simulink model "temp_regler"  (R2024a)
settings: Solver=VariableStepAuto  StartTime=0.0  StopTime=4200  RelTol=1e-3
values from neighbouring files (symbols this model uses):
  param_k1 = 10/400    (= 0.025)    [temp_regler.m]    (also in temp_regler_settings.m; temp_settings.m)
  param_k2 = 400/230    (= 1.73913043478)    [temp_regler.m]    (also in temp_regler_settings.m; temp_settings.m)
  param_switch_off = -0.2    [temp_regler.m]    (also in temp_regler_settings.m; temp_settings.m)
  param_switch_on = 0.2    [temp_regler.m]    (also in temp_regler_settings.m; temp_settings.m)
  param_time_const = 15*60    (= 900)    [temp_regler.m]    (also in temp_regler_settings.m; temp_settings.m)
settings Model: Creator=janho  LastModifiedBy=janho

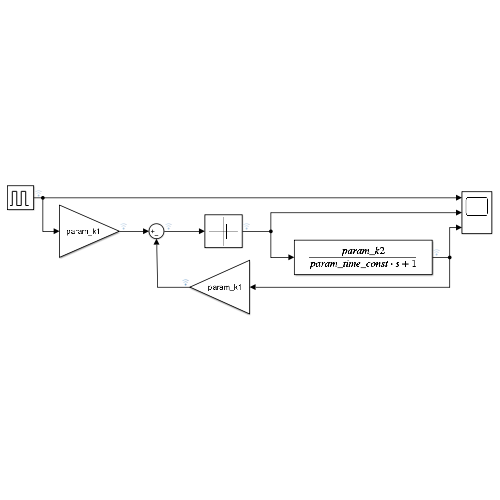
[thumbnail: Simulink's stored preview of the top-level diagram]
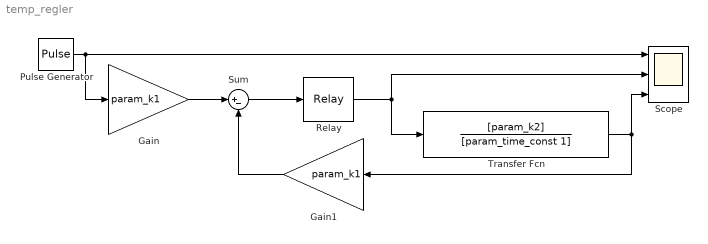
== system temp_regler ==
  Gain : Gain  Gain=param_k1
  Gain1 : Gain  Gain=param_k1
  Pulse Generator : DiscretePulseGenerator  PulseType=Time based  Amplitude=160  Period=70*60  PulseWidth=42.8
  Relay : Relay  OnSwitchValue=param_switch_on  OffSwitchValue=param_switch_off  OnOutputValue=param_switch_maxv  ZeroCross=off
  Scope : Scope  NumInputPorts=3
  Sum : Sum  Inputs=|+-
  Transfer Fcn : TransferFcn  Numerator=[param_k2]  Denominator=[param_time_const 1]
  wires:
  Relay/1 -> Scope/2, Transfer Fcn/1
  Gain1/1 -> Sum/2
  Gain/1 -> Sum/1
  Pulse Generator/1 -> Scope/1, Gain/1
  Sum/1 -> Relay/1
  Transfer Fcn/1 -> Scope/3, Gain1/1
